simulink model "Brk_Unit"  (R2020b)
settings: configuration reference "unit_config" (kept outside this file)
undefined symbols (not defined in the file): Ts
libraries: simulink_extras x1
settings Model: DataDictionary=Hybrid_vehicle.sldd  SimulationMode=accelerator  OrderedModelArguments=off  Creator=Georg  LastModifiedBy=jy
settings ConfigSetRef: SourceName=unit_config

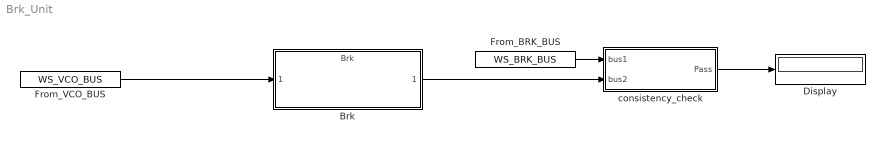
== system Brk_Unit ==
  Brk : ModelReference  ModelNameDialog=Brk  SimulationMode=Normal  ModelReferenceVersion=2.29
  Display : Display
  From_BRK_BUS : FromWorkspace  VariableName=WS_BRK_BUS  OutDataTypeStr=Bus: BRK_BUS  SampleTime=Ts  Interpolate=off  OutputAfterFinalValue=Holding final value
  From_VCO_BUS : FromWorkspace  VariableName=WS_VCO_BUS  OutDataTypeStr=Bus: VCO_BUS  SampleTime=Ts  Interpolate=off  OutputAfterFinalValue=Holding final value
  consistency_check : Subsystem
  wires:
  From_VCO_BUS/1 -> Brk/1
  From_BRK_BUS/1 -> consistency_check/1(bus1)
  Brk/1 -> consistency_check/2(bus2)
  consistency_check/1(Pass) -> Display/1

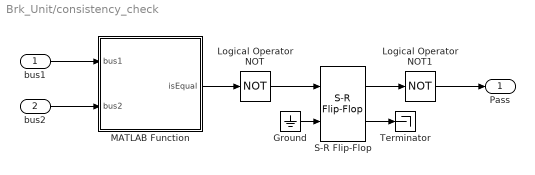
== system Brk_Unit/consistency_check ==
  bus1 : Inport
  bus2 : Inport  Port=2
  Ground : Ground
  Logical Operator NOT : Logic  Operator=NOT  AllPortsSameDT=off  OutDataTypeStr=boolean
  Logical Operator NOT1 : Logic  Operator=NOT  AllPortsSameDT=off  OutDataTypeStr=boolean
  MATLAB Function : MATLAB Function  TreatAsAtomicUnit=on
  S-R Flip-Flop : simulink_extras/Flip Flops/S-R Flip-Flop  initial_condition=0
  Terminator : Terminator
  Pass : Outport
  wires:
  bus1/1 -> MATLAB Function/1(bus1)
  bus2/1 -> MATLAB Function/2(bus2)
  MATLAB Function/1(isEqual) -> Logical Operator NOT/1
  Logical Operator NOT/1 -> S-R Flip-Flop/1
  Ground/1 -> S-R Flip-Flop/2
  S-R Flip-Flop/2 -> Terminator/1
  S-R Flip-Flop/1 -> Logical Operator NOT1/1
  Logical Operator NOT1/1 -> Pass/1

== matlab function Brk_Unit/consistency_check/MATLAB Function ==
  data: bus1 input; isEqual output; bus2 input
function isEqual = fcn(bus1, bus2)
isEqual = isequal(bus1, bus2);
